simulink model "boatx006_3"  (R2016a)
settings: Solver=ode4  StartTime=0.0  StopTime=20  FixedStep=0.01  RelTol=1e-3
values from neighbouring files (symbols this model uses):
  A = 5    [sm_boat_runx006_3.m]
  a1 = 1    [sm_boat_runx006_3.m]
  a2 = 1    [sm_boat_runx006_3.m]
  a3 = 1    [sm_boat_runx006_3.m]
  B = 30    [sm_boat_runx006_3.m]
  bmax = pi*(0.47)    (= 1.47654854719)    [sm_boat_runx006_3.m]
  d1 = 14    [sm_boat_runx006_3.m]
  d2 = 80    [sm_boat_runx006_3.m]
  d3 = 5    [sm_boat_runx006_3.m]
  fixedstep = 0.01    [sm_boat_runx006_3.m]
  Fmax = 20    [sm_boat_runx006_3.m]
  I = m*(W^2+L^2)/12    (= 0.759791666667)    [sm_boat_runx006_3.m]
  Izz = (0.1*m*W^2+1000*pi*D^2*L^3)/2/12    (= 0.336072151416)    [sm_boat_runx006_3.m]
  kai = pi*3/4    (= 2.35619449019)    [sm_boat_runx006_3.m]
  Lt = 0.4    [sm_boat_runx006_3.m]
  m = 7    [sm_boat_runx006_3.m]
  mxx = 0.05*m    (= 0.35)    [sm_boat_runx006_3.m]
  myy = 1000*pi*D^2*L/2    (= 3.92699081699)    [sm_boat_runx006_3.m]
  td = 0    [sm_boat_runx006_3.m]
  wd = fd*2*pi    (= 1.25663706144)    [sm_boat_runx006_3.m]
  wp_sh = 10    [sm_boat_runx006_3.m]
  wp_tol = 2.5    [sm_boat_runx006_3.m]
  Xw = R*cosd(ad)    [sm_boat_runx006_3.m]
  Yw = R*sind(ad)    [sm_boat_runx006_3.m]
libraries: simulink x1
settings Model: Creator=huangy  LastModifiedBy=huangy
settings DataIOCC: LimitDataPoints=on  SaveFormat=Array
settings HardwareCC: ProdBitPerPointer=32  ProdLargestAtomicFloat=None  ProdIntDivRoundTo=Undefined  ProdEndianess=Unspecified  ProdWordSize=32  ProdHWDeviceType=32-bit Generic
settings ModelReferenceCC: PropagateSignalLabelsOutOfModel=off
settings ConfigComp: CovModelRefEnable=Off
settings ConfigurationSet: Description=SimMechanics 2G

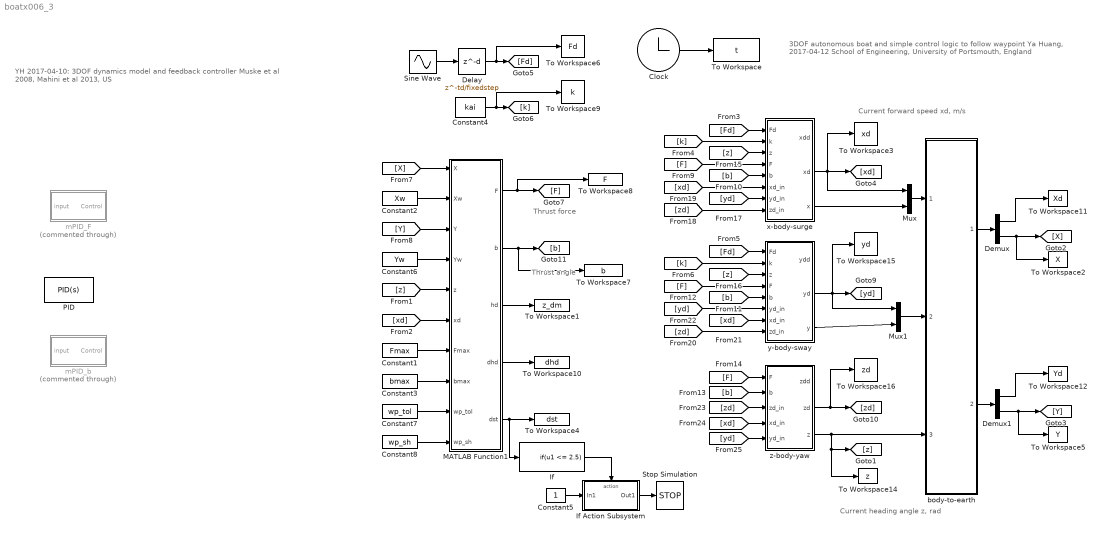
== system boatx006_3 ==
  note: 3DOF autonomous boat and simple control logic to follow waypoint
      | Ya Huang, 2017-04-12
      | School of Engineering, University of Portsmouth, England
  note: Thrust force
  note: Thrust angle
  note: Current heading angle z, rad
  note: Current forward speed xd, m/s
  note: YH 2017-04-10:
      | 3DOF dynamics model and feedback controller
      | Muske et al 2008, Mahini et al 2013, US
  Clock : Clock
  Constant1 : Constant  Value=Fmax  VectorParams1D=off
  Constant2 : Constant  Value=Xw  VectorParams1D=off
  Constant3 : Constant  Value=bmax  VectorParams1D=off
  Constant4 : Constant  Value=kai
  Constant5 : Constant  VectorParams1D=off
  Constant6 : Constant  Value=Yw  VectorParams1D=off
  Constant7 : Constant  Value=wp_tol  VectorParams1D=off
  Constant8 : Constant  Value=wp_sh  VectorParams1D=off
  Delay : Delay  DelayLength=td/fixedstep  InitialCondition=0
  Demux : Demux  Outputs=2
  Demux1 : Demux  Outputs=2
  If : If  IfExpression=u1 <= 2.5  ShowElse=off
  If Action Subsystem : Subsystem  TreatAsAtomicUnit=on
  MATLAB Function1 : MATLAB Function  TreatAsAtomicUnit=on
  Mux : Mux  Inputs=2
  Mux1 : Mux  Inputs=2
  PID : simulink/Continuous/PID Controller  Controller=PID  TimeDomain=Continuous-time  SampleTime=-1  IntegratorMethod=Forward Euler  FilterMethod=Forward Euler  Form=Parallel  UseFilter=on  ControllerParametersSource=internal  P=10  I=2  D=5  N=100  InitialConditionSource=internal  InitialConditionForIntegrator=0  InitialConditionForFilter=0  ExternalReset=none  LimitOutput=off  UpperSaturationLimit=inf  LowerSaturationLimit=-inf  LinearizeAsGain=on  AntiWindupMode=none  Kb=1  TrackingMode=off  Kt=1  PParamMin=[]  PParamMax=[]  IParamMin=[]  IParamMax=[]  DParamMin=[]  DParamMax=[]  NParamMin=[]  NParamMax=[]  KbParamMin=[]  KbParamMax=[]  KtParamMin=[]  KtParamMax=[]  POutMin=[]  POutMax=[]  IOutMin=[]  IOutMax=[]  DOutMin=[]  DOutMax=[]  NOutMin=[]  NOutMax=[]  KbOutMin=[]  KbOutMax=[]  KtOutMin=[]  KtOutMax=[]  IntegratorOutMin=[]  IntegratorOutMax=[]  FilterOutMin=[]  FilterOutMax=[]  SumOutMin=[]  SumOutMax=[]  SumI1OutMin=[]  SumI1OutMax=[]  SumI2OutMin=[]  SumI2OutMax=[]  SumI3OutMin=[]  SumI3OutMax=[]  SumDOutMin=[]  SumDOutMax=[]  SaturationOutMin=[]  SaturationOutMax=[]  IntegratorContinuousStateAttributes=''  IntegratorStateMustResolveToSignalObject=off  IntegratorRTWStateStorageClass=Auto  FilterContinuousStateAttributes=''  FilterStateMustResolveToSignalObject=off  FilterRTWStateStorageClass=Auto  DifferentiatorICPrevScaledInput=0  DifferentiatorOutMin=[]  DifferentiatorOutMax=[]
  Sine Wave : Sin  Amplitude=A  Bias=B  Frequency=wd  SampleTime=0
  Stop Simulation : Stop
  To Workspace : ToWorkspace  VariableName=t  SaveFormat=Timeseries  SampleTime=-1
  To Workspace1 : ToWorkspace  VariableName=z_dm  SaveFormat=Timeseries  SampleTime=-1
  To Workspace10 : ToWorkspace  VariableName=dhd  SaveFormat=Timeseries  SampleTime=-1
  To Workspace11 : ToWorkspace  VariableName=Xd  SaveFormat=Timeseries  SampleTime=-1
  To Workspace12 : ToWorkspace  VariableName=Yd  SaveFormat=Timeseries  SampleTime=-1
  To Workspace14 : ToWorkspace  VariableName=z  SaveFormat=Timeseries  SampleTime=-1
  To Workspace15 : ToWorkspace  VariableName=yd  SaveFormat=Timeseries  SampleTime=-1
  To Workspace16 : ToWorkspace  VariableName=zd  SaveFormat=Timeseries  SampleTime=-1
  To Workspace2 : ToWorkspace  VariableName=X  SaveFormat=Timeseries  SampleTime=-1
  To Workspace3 : ToWorkspace  VariableName=xd  SaveFormat=Timeseries  SampleTime=-1
  To Workspace4 : ToWorkspace  VariableName=dst  SaveFormat=Timeseries  SampleTime=-1
  To Workspace5 : ToWorkspace  VariableName=Y  SaveFormat=Timeseries  SampleTime=-1
  To Workspace6 : ToWorkspace  VariableName=Fd  SaveFormat=Timeseries  SampleTime=-1
  To Workspace7 : ToWorkspace  VariableName=b  SaveFormat=Timeseries  SampleTime=-1
  To Workspace8 : ToWorkspace  VariableName=F  SaveFormat=Timeseries  SampleTime=-1
  To Workspace9 : ToWorkspace  VariableName=k  SaveFormat=Timeseries  SampleTime=-1
  body-to-earth : Subsystem
  mPID_F : Subsystem  Commented=through  mask{kp=5, ki=2, kd=0}
  mPID_b : Subsystem  Commented=through  mask{kp=5, ki=2, kd=10}
  x-body-surge : Subsystem
  y-body-sway : Subsystem
  z-body-yaw : Subsystem
  wires:
  Clock/1 -> To Workspace/1
  z-body-yaw/2(zd) -> To Workspace16/1, [zd]
  [X] -> MATLAB Function1/1(X)
  [Y] -> MATLAB Function1/3(Y)
  Constant6/1 -> MATLAB Function1/4(Yw)
  Constant2/1 -> MATLAB Function1/2(Xw)
  [z] -> MATLAB Function1/5(z)
  Constant1/1 -> MATLAB Function1/7(Fmax)
  Constant3/1 -> MATLAB Function1/8(bmax)
  MATLAB Function1/3(hd) -> To Workspace1/1
  [xd] -> MATLAB Function1/6(xd)
  MATLAB Function1/5(dst) -> To Workspace4/1, If/1
  Constant4/1 -> To Workspace9/1, [k]
  [Fd] -> x-body-surge/1(Fd)
  [k] -> x-body-surge/2(k)
  [Fd] -> y-body-sway/1(Fd)
  [k] -> y-body-sway/2(k)
  [F] -> x-body-surge/4(F)
  [b] -> x-body-surge/5(b)
  [b] -> y-body-sway/5(b)
  [F] -> y-body-sway/4(F)
  [F] -> z-body-yaw/1(F)
  [b] -> z-body-yaw/2(b)
  x-body-surge/2(xd) -> Mux/1, [xd], To Workspace3/1
  [z] -> x-body-surge/3(z)
  [z] -> y-body-sway/3(z)
  Sine Wave/1 -> Delay/1
  Delay/1 -> [Fd], To Workspace6/1
  If/1 -> If Action Subsystem/Action
  If Action Subsystem/1(Out1) -> Stop Simulation/1
  Constant5/1 -> If Action Subsystem/1(In1)
  Constant7/1 -> MATLAB Function1/9(wp_tol)
  Constant8/1 -> MATLAB Function1/10(wp_sh)
  MATLAB Function1/4(dhd) -> To Workspace10/1
  MATLAB Function1/1(F) -> To Workspace8/1, [F]
  [yd] -> x-body-surge/7(yd_in)
  y-body-sway/2(yd) -> To Workspace15/1, [yd], Mux1/1
  [zd] -> x-body-surge/8(zd_in)
  [xd] -> x-body-surge/6(xd_in)
  [yd] -> y-body-sway/6(yd_in)
  [zd] -> y-body-sway/8(zd_in)
  [xd] -> y-body-sway/7(xd_in)
  [zd] -> z-body-yaw/3(zd_in)
  [xd] -> z-body-yaw/4(xd_in)
  [yd] -> z-body-yaw/5(yd_in)
  Mux/1 -> body-to-earth/1(x_body)
  x-body-surge/3(x) -> Mux/2
  y-body-sway/3(y) -> Mux1/2
  Mux1/1 -> body-to-earth/2(y_body)
  z-body-yaw/3(z) -> body-to-earth/3(z_yaw angle), [z], To Workspace14/1
  body-to-earth/1(X_earth) -> Demux/1
  body-to-earth/2(Y_earth) -> Demux1/1
  Demux1/2 -> To Workspace5/1, [Y]
  Demux/2 -> To Workspace2/1, [X]
  Demux/1 -> To Workspace11/1
  Demux1/1 -> To Workspace12/1
  MATLAB Function1/2(b) -> [b], To Workspace7/1

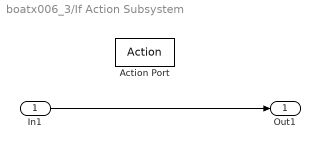
== system boatx006_3/If Action Subsystem ==
  In1 : Inport
  Action Port : ActionPort  ActionType=then
  Out1 : Outport
  wires:
  In1/1 -> Out1/1

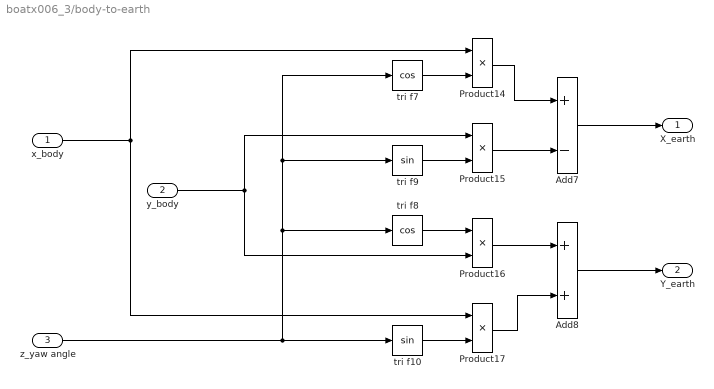
== system boatx006_3/body-to-earth ==
  x_body : Inport
  y_body : Inport  Port=2
  z_yaw angle : Inport  Port=3
  Add7 : Sum  Inputs=+-
  Add8 : Sum
  Product{14..17} (4 alike) : Product
  tri f10 : Trigonometry
  tri f7 : Trigonometry  Operator=cos
  tri f8 : Trigonometry  Operator=cos
  tri f9 : Trigonometry
  X_earth : Outport
  Y_earth : Outport  Port=2
  wires:
  tri f7/1 -> Product14/2
  tri f10/1 -> Product17/2
  y_body/1 -> Product16/2, Product15/1
  tri f9/1 -> Product15/2
  Add7/1 -> X_earth/1
  tri f8/1 -> Product16/1
  Product17/1 -> Add8/2
  Product15/1 -> Add7/2
  Add8/1 -> Y_earth/1
  Product16/1 -> Add8/1
  Product14/1 -> Add7/1
  z_yaw angle/1 -> tri f7/1, tri f9/1, tri f8/1, tri f10/1
  x_body/1 -> Product17/1, Product14/1

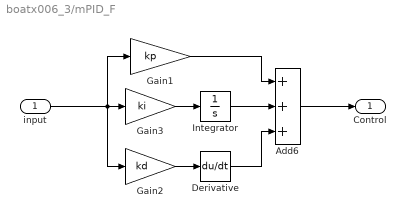
== system boatx006_3/mPID_F ==
  input : Inport
  Add6 : Sum  Inputs=+++
  Derivative : Derivative
  Gain1 : Gain  Gain=kp
  Gain2 : Gain  Gain=kd
  Gain3 : Gain  Gain=ki
  Integrator : Integrator
  Control : Outport
  wires:
  input/1 -> Gain1/1, Gain2/1, Gain3/1
  Gain1/1 -> Add6/1
  Gain2/1 -> Derivative/1
  Derivative/1 -> Add6/3
  Gain3/1 -> Integrator/1
  Integrator/1 -> Add6/2
  Add6/1 -> Control/1

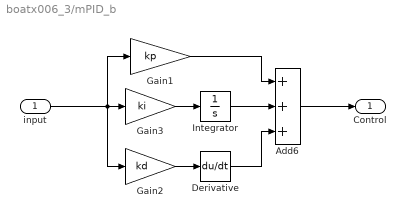
== system boatx006_3/mPID_b ==
  input : Inport
  Add6 : Sum  Inputs=+++
  Derivative : Derivative
  Gain1 : Gain  Gain=kp
  Gain2 : Gain  Gain=kd
  Gain3 : Gain  Gain=ki
  Integrator : Integrator
  Control : Outport
  wires:
  input/1 -> Gain1/1, Gain2/1, Gain3/1
  Gain1/1 -> Add6/1
  Gain2/1 -> Derivative/1
  Derivative/1 -> Add6/3
  Gain3/1 -> Integrator/1
  Integrator/1 -> Add6/2
  Add6/1 -> Control/1

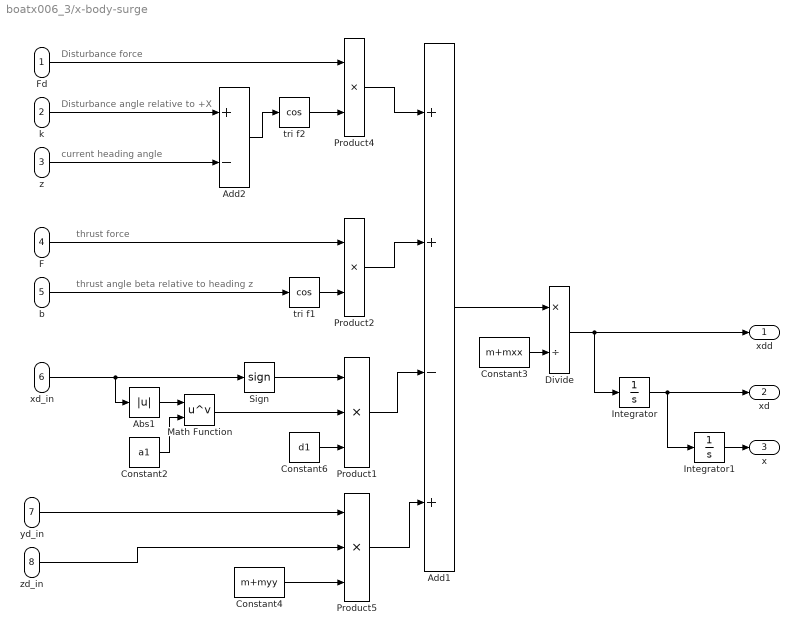
== system boatx006_3/x-body-surge ==
  note: current heading angle
  note: thrust force
  note: thrust angle beta relative to heading z
  note: Disturbance force
  note: Disturbance angle relative to +X
  Fd : Inport
  k : Inport  Port=2
  z : Inport  Port=3
  F : Inport  Port=4
  b : Inport  Port=5
  xd_in : Inport  Port=6
  yd_in : Inport  Port=7
  zd_in : Inport  Port=8
  Abs1 : Abs
  Add1 : Sum  Inputs=++-+
  Add2 : Sum  Inputs=+-
  Constant2 : Constant  Value=a1
  Constant3 : Constant  Value=m+mxx  VectorParams1D=off
  Constant4 : Constant  Value=m+myy  VectorParams1D=off
  Constant6 : Constant  Value=d1
  Divide : Product  Inputs=*/
  Integrator : Integrator
  Integrator1 : Integrator
  Math Function : Math  Operator=pow  SaturateOnIntegerOverflow=on
  Product1 : Product  Inputs=3
  Product2 : Product
  Product4 : Product
  Product5 : Product  Inputs=3
  Sign : Signum
  tri f1 : Trigonometry  Operator=cos
  tri f2 : Trigonometry  Operator=cos
  xdd : Outport
  xd : Outport  Port=2
  x : Outport  Port=3
  wires:
  xd_in/1 -> Sign/1, Abs1/1
  tri f1/1 -> Product2/2
  b/1 -> tri f1/1
  F/1 -> Product2/1
  Integrator/1 -> xd/1, Integrator1/1
  Integrator1/1 -> x/1
  Add1/1 -> Divide/1
  Constant3/1 -> Divide/2
  Divide/1 -> Integrator/1, xdd/1
  Product4/1 -> Add1/1
  tri f2/1 -> Product4/2
  Fd/1 -> Product4/1
  Product2/1 -> Add1/2
  Add2/1 -> tri f2/1
  k/1 -> Add2/1
  z/1 -> Add2/2
  Product5/1 -> Add1/4
  yd_in/1 -> Product5/1
  zd_in/1 -> Product5/2
  Constant4/1 -> Product5/3
  Product1/1 -> Add1/3
  Abs1/1 -> Math Function/1
  Constant2/1 -> Math Function/2
  Math Function/1 -> Product1/2
  Constant6/1 -> Product1/3
  Sign/1 -> Product1/1

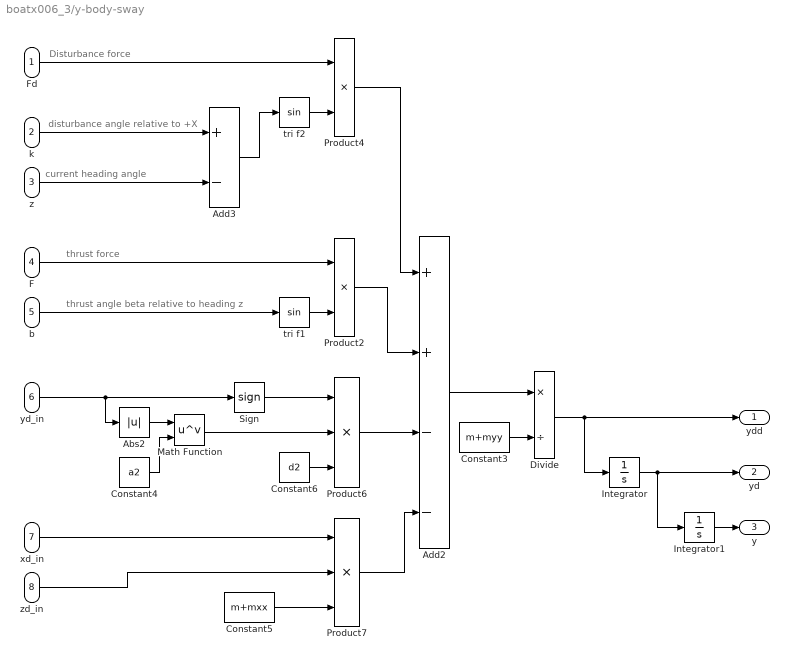
== system boatx006_3/y-body-sway ==
  note: thrust force
  note: thrust angle beta relative to heading z
  note: Disturbance force
  note: current heading angle
  note: disturbance angle relative to +X
  Fd : Inport
  k : Inport  Port=2
  z : Inport  Port=3
  F : Inport  Port=4
  b : Inport  Port=5
  yd_in : Inport  Port=6
  xd_in : Inport  Port=7
  zd_in : Inport  Port=8
  Abs2 : Abs
  Add2 : Sum  Inputs=++--
  Add3 : Sum  Inputs=+-
  Constant3 : Constant  Value=m+myy  VectorParams1D=off
  Constant4 : Constant  Value=a2
  Constant5 : Constant  Value=m+mxx  VectorParams1D=off
  Constant6 : Constant  Value=d2
  Divide : Product  Inputs=*/
  Integrator : Integrator
  Integrator1 : Integrator
  Math Function : Math  Operator=pow  SaturateOnIntegerOverflow=on
  Product2 : Product
  Product4 : Product
  Product6 : Product  Inputs=3
  Product7 : Product  Inputs=3
  Sign : Signum
  tri f1 : Trigonometry
  tri f2 : Trigonometry
  ydd : Outport
  yd : Outport  Port=2
  y : Outport  Port=3
  wires:
  Product2/1 -> Add2/2
  tri f1/1 -> Product2/2
  b/1 -> tri f1/1
  Integrator/1 -> yd/1, Integrator1/1
  Integrator1/1 -> y/1
  F/1 -> Product2/1
  Add2/1 -> Divide/1
  Constant3/1 -> Divide/2
  Divide/1 -> Integrator/1, ydd/1
  Product4/1 -> Add2/1
  tri f2/1 -> Product4/2
  Fd/1 -> Product4/1
  k/1 -> Add3/1
  z/1 -> Add3/2
  Add3/1 -> tri f2/1
  yd_in/1 -> Sign/1, Abs2/1
  Product7/1 -> Add2/4
  xd_in/1 -> Product7/1
  zd_in/1 -> Product7/2
  Constant5/1 -> Product7/3
  Product6/1 -> Add2/3
  Abs2/1 -> Math Function/1
  Constant4/1 -> Math Function/2
  Math Function/1 -> Product6/2
  Constant6/1 -> Product6/3
  Sign/1 -> Product6/1

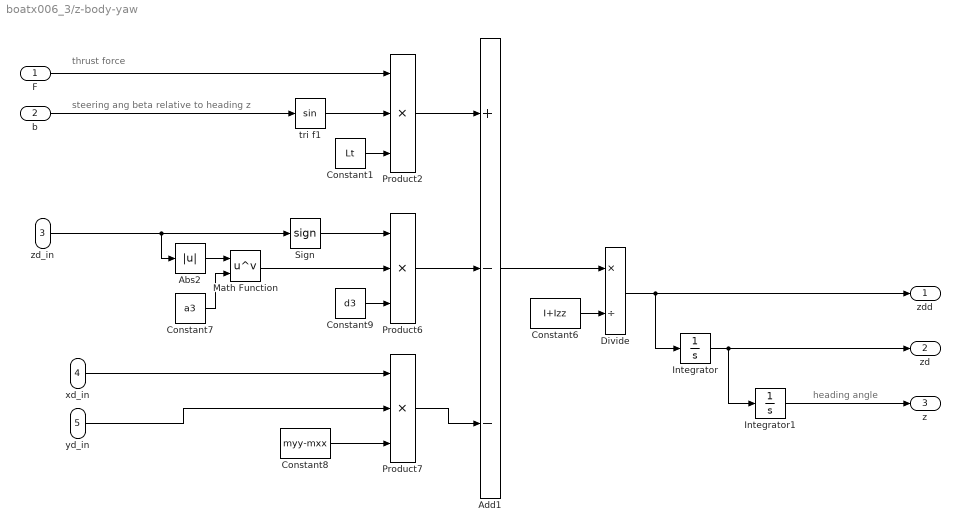
== system boatx006_3/z-body-yaw ==
  note: heading angle
  note: thrust force
  note: steering ang beta relative to heading z
  F : Inport
  b : Inport  Port=2
  zd_in : Inport  Port=3
  xd_in : Inport  Port=4
  yd_in : Inport  Port=5
  Abs2 : Abs
  Add1 : Sum  Inputs=+--
  Constant1 : Constant  Value=Lt
  Constant6 : Constant  Value=I+Izz  VectorParams1D=off
  Constant7 : Constant  Value=a3
  Constant8 : Constant  Value=myy-mxx  VectorParams1D=off
  Constant9 : Constant  Value=d3
  Divide : Product  Inputs=*/
  Integrator : Integrator
  Integrator1 : Integrator
  Math Function : Math  Operator=pow  SaturateOnIntegerOverflow=on
  Product2 : Product  Inputs=3
  Product6 : Product  Inputs=3
  Product7 : Product  Inputs=3
  Sign : Signum
  tri f1 : Trigonometry
  zdd : Outport
  zd : Outport  Port=2
  z : Outport  Port=3
  wires:
  F/1 -> Product2/1
  tri f1/1 -> Product2/2
  b/1 -> tri f1/1
  Product2/1 -> Add1/1
  Constant1/1 -> Product2/3
  Integrator/1 -> zd/1, Integrator1/1
  Integrator1/1 -> z/1
  Add1/1 -> Divide/1
  Constant6/1 -> Divide/2
  Divide/1 -> Integrator/1, zdd/1
  zd_in/1 -> Sign/1, Abs2/1
  Product7/1 -> Add1/3
  xd_in/1 -> Product7/1
  yd_in/1 -> Product7/2
  Constant8/1 -> Product7/3
  Product6/1 -> Add1/2
  Abs2/1 -> Math Function/1
  Constant7/1 -> Math Function/2
  Math Function/1 -> Product6/2
  Constant9/1 -> Product6/3
  Sign/1 -> Product6/1

== matlab function boatx006_3/MATLAB Function1 ==
  data: F output; b output; X input; Xw input; Y input; Yw input; z input; xd input; Fmax input; bmax input; hd output; dhd output; dst output; wp_tol input; wp_sh input
function [F,b,hd,dhd,dst] = nav(X,Xw,Y,Yw,z,xd,Fmax,bmax,wp_tol,wp_sh)
% #codegen
% Xw Yw - m, current waypoint
% X Y - m, current position
% z - rad, current heading
% V - m/s, forward speed demand
% Fmax - N, max thrust force 
% b - rad, max thruster steer angle demand
% YH 2017-03-25

Xdiff = Xw - X ; % m, X position error
Ydiff = Yw - Y ;
dst = sqrt(Xdiff^2 + Ydiff^2) ; % m, distance to next waypoint

hd = atan2(Ydiff,Xdiff) ; % rad, heading demand by calculation
% atan2(y,x) returns 4 quadrant inverse tangent in range [-pi, pi]
dhd = hd - z ; % rad, different between demand and current heading

F = 0 ;
b = 0 ;

if dhd < -pi % negative heading difference too large
    dhd = 2*pi + hd - z ; % add 2*pi to avoid swirl
    hd = 2*pi + hd ; % to display the corrected hd
elseif dhd > pi % positive heading difference too large
    dhd = -2*pi + hd - z ; % add -2*pi to avoid swirl
    hd = -2*pi + hd ; % corrected hd
end

if (dst <= wp_tol) % close to waypoint
    F = 0 ; % stop engine
    b = 0 ;
else
    if (dhd > -pi/2) && (dhd < pi/2) % heading difference small
%         b = bmax*dhd/(pi/2) ; % thruster angle proportional to heading difference
        b = bmax*dhd/(pi/2) ; % thruster angle proportional to heading difference
        F = Fmax ;
    elseif ((dhd >= -pi)&&(dhd <= -pi/2)) || ((dhd >= pi/2)&&(dhd <= pi)) % heading difference large
        b = bmax*(sign(dhd)) ; % thruster angle maximum
        if (dst <= wp_sh) % remaining distance too short for turn at large heading difference 
            F = (Fmax/3)*(dst/wp_sh) ; % thrust proportional to distance and limited to a third of max
        else
            F = Fmax/2 ; % thrust limited to half max
        end
    end
end

% if (Xdiff>0)&&(Ydiff>0) % 1st quadrant
%     hd_rad = atan(Ydiff/Xdiff) ;
% elseif (Xdiff>0)&&(Ydiff<0) % 4th quadrant
%     hd_rad = atan(Ydiff/Xdiff) ;
% elseif (Xdiff<0)&&(Ydiff>0) % 2nd quadrant 
%     hd_rad = pi + atan(Ydiff/Xdiff) ;
% elseif (Xdiff<0)&&(Ydiff<0) % 3rd quadrant
%     hd_rad = -pi + atan(Ydiff/Xdiff) ;
% end

% if (Xdiff>0.01) && (Ydiff>0.01) % 1st quadrant
%     hd_rad = atan(Ydiff/Xdiff) ;
% elseif (Xdiff>0.01) && (Ydiff<-0.01) % 4th quadrant
%     hd_rad = atan(Ydiff/Xdiff) ;
% elseif (Xdiff<-0.01) && (Ydiff>0.01) % 2nd quadrant 
%     hd_rad = pi + atan(Ydiff/Xdiff) ;
% elseif (Xdiff<-0.01) && (Ydiff<-0.01) % 3rd quadrant
%     hd_rad = -pi + atan(Ydiff/Xdiff) ;
% elseif (-0.01<=Xdiff<=0.01) && (Ydiff>=0.01) % when reaching Xw not Yw
%     hd_rad = pi/2 ; 
% elseif (-0.01<=Xdiff<=0.01) && (Ydiff<=-0.01)
%     hd_rad = -pi/2 ;
% elseif (Xdiff>=0.01) && (-0.01<=Ydiff<=0.01) % when reaching Yw not Xw
%     hd_rad = 0 ;
% elseif (Xdiff<=-0.01) && (-0.01<=Ydiff<=0.01)
%     hd_rad = pi ;
% end
